simulink model "test_environment"  (R2016a)
settings: Solver=VariableStepAuto  StartTime=0.0  StopTime=10.0  RelTol=1e-3
libraries: vrlib x1
settings Model: Creator=jcfinnerup  LastModifiedBy=jcfinnerup

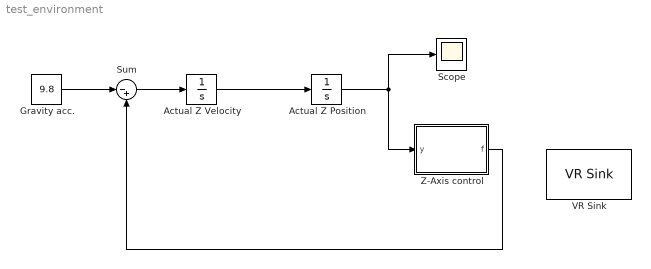
== system test_environment ==
  Actual Z Position : Integrator  InitialCondition=20  LimitOutput=on  LowerSaturationLimit=0
  Actual Z Velocity : Integrator
  Gravity acc. : Constant  Value=9.8
  Scope : Scope
  Sum : Sum  Inputs=|-+
  VR Sink : vrlib/VR Sink  InstantiateOnLoad=on  SampleTime=0.1  ViewEnable=on  RemoteChange=off  RemoteView=off  WorldFileName=VR3D/environment.wrl  AutoView=off  VideoDimensions=[]  AllowVariableSize=off
  Z-Axis control : MATLAB Function  TreatAsAtomicUnit=on
  wires:
  Gravity acc./1 -> Sum/1
  Actual Z Velocity/1 -> Actual Z Position/1
  Sum/1 -> Actual Z Velocity/1
  Actual Z Position/1 -> Z-Axis control/1(y), Scope/1
  Z-Axis control/1(f) -> Sum/2

== matlab function test_environment/Z-Axis control ==
  data: y input; f output


function f = fcn(y)

% Always returns 0
f = 0*y;
